simulink model "mod5_counter"  (R2020b)
settings: Solver=VariableStepAuto  StartTime=0.0  StopTime=10.0  RelTol=1e-3
settings Model: Creator=Vrunda M Balgi  LastModifiedBy=Vrunda M Balgi

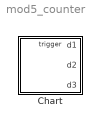
== system mod5_counter ==
  Chart : Stateflow chart  TreatAsAtomicUnit=on

== stateflow chart mod5_counter/Chart ==
  state digit1 [parallel]
    settings: executionOrder=1
    state Zero
      entry:
      d1 = 0;
    state One
      entry:
      d1 = 1;
    (default) -> digit1.Zero
    digit1.Zero -> digit1.One : input_trigger
    digit1.One -> digit1.Zero : input_trigger
  state digit2 [parallel]
    settings: executionOrder=2
    state Zero
      entry:
      d2 = 0;
    state One
      entry:
      d2 = 1;
    (default) -> digit2.Zero
    digit2.Zero -> digit2.One
    digit2.One -> digit2.Zero
  state digit3 [parallel]
    settings: executionOrder=3
    state Zero
      entry:
      d3 = 0;
    state One
      entry:
      d3 = 1;
    (default) -> digit3.Zero
    digit3.Zero -> digit3.One
    digit3.One -> digit3.Zero
  data: d1 output; d2 output; d3 output
  events: local_it2 local FUNCTION_CALL_EVENT; local_it3 local FUNCTION_CALL_EVENT; input_trigger input FUNCTION_CALL_EVENT
